simulink model "testBCIRobot"  (Simulink 10.0)
settings: Solver=FixedStepDiscrete  StartTime=0.0  StopTime=inf  FixedStep=0.002  MaxStep=0.02  RelTol=1e-3  AbsTol=1e-6
settings Model: Creator=fwornle  LastModifiedBy=bhisma  ExtModeTrigDuration=5000
settings ConfigSet: Description=rtmc9s12target_R2009b
settings SolverCC: AutoScaleAbsTol=off
settings DataIOCC: SignalLoggingSaveFormat=ModelDataLogs  SaveOutput=off  SaveTime=off  SignalLoggingName=sigsOut
settings OptimizationCC: BlockReduction=off  BooleanDataType=off  ExpressionDepthLimit=2147483647  InitFltsAndDblsToZero=on  LifeSpan=1  EfficientTunableParamExpr=on
settings DebuggingCC: SaveWithParameterizedLinksMsg=none  SignalResolutionControl=TryResolveAllWithWarning  MultiTaskDSMMsg=warning  MultiTaskCondExecSysMsg=none  FcnCallInpInsideContextMsg=warning  StateNameClashWarn=warning
settings HardwareCC: ProdBitPerInt=16  ProdBitPerPointer=16  ProdBitPerSizeT=16  ProdBitPerPtrDiffT=16  ProdEndianess=BigEndian  ProdWordSize=16  ProdHWDeviceType=Motorola HC12
settings SFSimCC: MATLABDynamicMemAlloc=off
settings RTWCC: SystemTargetFile=mc9s12.tlc  GenerateMakefile=off  TemplateMakefile=mc9s12.tmf
settings CodeAppCC: IgnoreCustomStorageClasses=off  CustomSymbolStrType=$N$R$M  InternalIdentifier=Classic
settings STFCustomTargetCC: TargetFcnLib=ansi_tfl_tmw.mat  ModelReferenceCompliant=off  IncludeMdlTerminateFcn=off  ERTCustomFileBanners=on  SupportNonInlinedSFcns=off  RemoveResetFunc=on  MATLABClassNameForMDSCustomization=Simulink.SoftwareTarget.ERTCustomization  CPPClassGenCompliant=on  SystemTargetFile=mc9s12.tlc
settings ERTTargetCC: TargetFcnLib=ansi_tfl_tmw.mat  MultiwordLength=2048  ModelReferenceCompliant=off  ParMdlRefBuildCompliant=off  CompOptLevelCompliant=off  ConcurrentExecutionCompliant=off  IncludeMdlTerminateFcn=off  CombineOutputUpdateFcns=off  SupportContinuousTime=on  ModelStepFunctionPrototypeControlCompliant=off  GRTInterface=on  UseToolchainInfoCompliant=off  ExtModeMexFile=ext_serial_mc9s12_comm  ExtModeMexArgs=1,2,115200  ERTCustomFileTemplate=mc9s12_file_process.tlc  ConvertIfToSwitch=off  SuppressUnreachableDefaultCases=off
settings CustomProperty: DataType=RTWOptions_EnumType_C__Users_fw__SVN_rtmc9s12-target_trunk_rtmc9s12_CW_R2009b_bin_mc9s12_1mc9s12_TargetBoard  Value=MiniDragonPlus-RevE
settings EnumStrPairs: String=Dragon12
settings ConfigComp: CovExternalEMLEnable=off

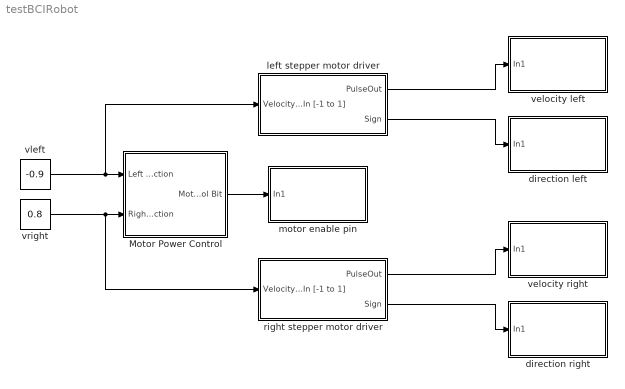
== system testBCIRobot ==
  Motor Power Control : Subsystem
  direction left : Subsystem  Tag=mcTarget_digOut  mask{port=Port A, pin=5, sampletime=0.002, Von=0.5, Voff=0.5}
      mask prompts: port "Port (see hardware manuals for valid options)"; pin "Pin (see hardware manuals for valid options)"; sampletime "Sample time"; Von "On-threshold (Von)"; Voff "Off-threshold (Voff)"
      mask init:
      | [portstr, pinstr, pins] = mbc_digitaloutput(port, pin, sampletime, Von, Voff);
      mask Help: web('digOut_sfcn_9S12.html');
      mask TypeOptions port: Port A | Port B | Port H | Port J | Port M | Port P | Port S | Port T
      mask Display: fprintf('%s\nPins: %s', portstr, pinstr)
  direction right : Subsystem  Tag=mcTarget_digOut  mask{port=Port A, pin=7, sampletime=0.002, Von=0.5, Voff=0.5}
      mask prompts: port "Port (see hardware manuals for valid options)"; pin "Pin (see hardware manuals for valid options)"; sampletime "Sample time"; Von "On-threshold (Von)"; Voff "Off-threshold (Voff)"
      mask init:
      | [portstr, pinstr, pins] = mbc_digitaloutput(port, pin, sampletime, Von, Voff);
      mask Help: web('digOut_sfcn_9S12.html');
      mask TypeOptions port: Port A | Port B | Port H | Port J | Port M | Port P | Port S | Port T
      mask Display: fprintf('%s\nPins: %s', portstr, pinstr)
  left stepper motor driver : Subsystem  mask{Nmax=200, Ninc=20, Ts=2e-3}
      mask prompts: Nmax "Maximum number of pulses per second (Nmax)"; Ninc "Number of increments (Ninc = 1 ... Nmax)"; Ts "Sample time"
      mask help: The block sample time (seconds) is used to clock the digital motor driver algorithm. Smaller values lead to slower pulse sequences.
      mask init:
      | Nmax = floor(abs(Nmax));
      | Ninc = max(1, floor(abs(Ninc)));
      | if (Ninc > Nmax)
      | 	error(['Stepper motor driver: Invalid number of increments (Ninc = ' num2str(Ninc) '; value must be smaller or equal to Nmax = ' num2str(Nmax) ')'])
      | end
      | 
      | % work out pulse length
      | Tpulse_ = 1/Nmax/2;
      | %disp(['Pulse length: ' num2str(1000*Tpulse_) ' ms.'])
      | 
      | % ensure that sample time is fixed multiple of 'Ts'
      | Tpulse = ceil(Tpulse_/Ts)*Ts;
      | if (Tpulse > Tpulse_)
      | 	disp('Decreasing maximum number of pulses per second to ensure that the pulse duration is an integer multiple of ''Ts''')
      | 	
      | 	% adjust Nmax
      | 	Nmax = floor(1/Tpulse/2);
      | 	disp(['New Nmax: ' num2str(Nmax) ' pulses per second.'])
      | end
      | 	
      | % work out quantization interval
      | dQ = floor(Nmax/Ninc);
  motor enable pin : Subsystem  Tag=mcTarget_digOut  mask{port=Port T, pin=7, sampletime=0.002, Von=0.5, Voff=0.5}
      mask prompts: port "Port (see hardware manuals for valid options)"; pin "Pin (see hardware manuals for valid options)"; sampletime "Sample time"; Von "On-threshold (Von)"; Voff "Off-threshold (Voff)"
      mask init:
      | [portstr, pinstr, pins] = mbc_digitaloutput(port, pin, sampletime, Von, Voff);
      mask Help: web('digOut_sfcn_9S12.html');
      mask TypeOptions port: Port A | Port B | Port H | Port J | Port M | Port P | Port S | Port T
      mask Display: fprintf('%s\nPins: %s', portstr, pinstr)
  right stepper motor driver : Subsystem  mask{Nmax=200, Ninc=20, Ts=2e-3}
      mask prompts: Nmax "Maximum number of pulses per second (Nmax)"; Ninc "Number of increments (Ninc = 1 ... Nmax)"; Ts "Sample time"
      mask help: The block sample time (seconds) is used to clock the digital motor driver algorithm. Smaller values lead to slower pulse sequences.
      mask init: same as testBCIRobot/left stepper motor driver
  velocity left : Subsystem  Tag=mcTarget_digOut  mask{port=Port A, pin=4, sampletime=0.002, Von=0.5, Voff=0.5}
      mask prompts: port "Port (see hardware manuals for valid options)"; pin "Pin (see hardware manuals for valid options)"; sampletime "Sample time"; Von "On-threshold (Von)"; Voff "Off-threshold (Voff)"
      mask init:
      | [portstr, pinstr, pins] = mbc_digitaloutput(port, pin, sampletime, Von, Voff);
      mask Help: web('digOut_sfcn_9S12.html');
      mask TypeOptions port: Port A | Port B | Port H | Port J | Port M | Port P | Port S | Port T
      mask Display: fprintf('%s\nPins: %s', portstr, pinstr)
  velocity right : Subsystem  Tag=mcTarget_digOut  mask{port=Port A, pin=6, sampletime=0.002, Von=0.5, Voff=0.5}
      mask prompts: port "Port (see hardware manuals for valid options)"; pin "Pin (see hardware manuals for valid options)"; sampletime "Sample time"; Von "On-threshold (Von)"; Voff "Off-threshold (Voff)"
      mask init:
      | [portstr, pinstr, pins] = mbc_digitaloutput(port, pin, sampletime, Von, Voff);
      mask Help: web('digOut_sfcn_9S12.html');
      mask TypeOptions port: Port A | Port B | Port H | Port J | Port M | Port P | Port S | Port T
      mask Display: fprintf('%s\nPins: %s', portstr, pinstr)
  vleft : Constant  Value=-0.9
  vright : Constant  Value=0.8
  wires:
  left stepper motor driver/1(PulseOut) -> velocity left/1(In1)
  left stepper motor driver/2(Sign) -> direction left/1(In1)
  right stepper motor driver/1(PulseOut) -> velocity right/1(In1)
  right stepper motor driver/2(Sign) -> direction right/1(In1)
  Motor Power Control/1(Motor Control Bit) -> motor enable pin/1(In1)
  vleft/1 -> Motor Power Control/1(Left Motor Instruction), left stepper motor driver/1(VelocityIn [-1 to 1])
  vright/1 -> Motor Power Control/2(Right Motor  Instruction), right stepper motor driver/1(VelocityIn [-1 to 1])

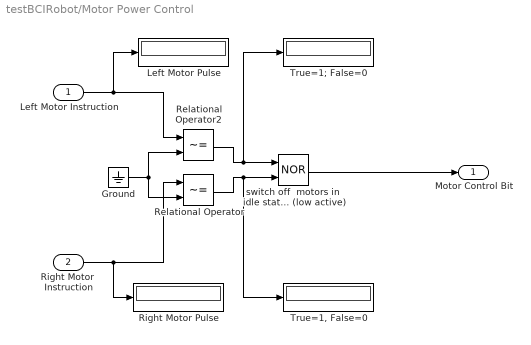
== system testBCIRobot/Motor Power Control ==
  Left Motor Instruction : Inport
  Right Motor  Instruction : Inport  Port=2
  Ground : Ground
  Left Motor Pulse : Display
  Relational Operator : RelationalOperator  Operator=~=  RndMeth=Nearest
  Relational Operator2 : RelationalOperator  Operator=~=  RndMeth=Nearest
  Right Motor Pulse : Display
  "True=1, False=0" : Display
  True=1; False=0 : Display
  switch off  motors in  idle state (low active) : Logic  Operator=NOR  AllPortsSameDT=off
  Motor Control Bit : Outport
  wires:
  Right Motor  Instruction/1 -> Relational Operator/1, Right Motor Pulse/1
  Left Motor Instruction/1 -> Relational Operator2/1, Left Motor Pulse/1
  Ground/1 -> Relational Operator2/2, Relational Operator/2
  Relational Operator2/1 -> switch off  motors in  idle state (low active)/1, True=1; False=0/1
  Relational Operator/1 -> switch off  motors in  idle state (low active)/2, "True=1, False=0"/1
  switch off  motors in  idle state (low active)/1 -> Motor Control Bit/1

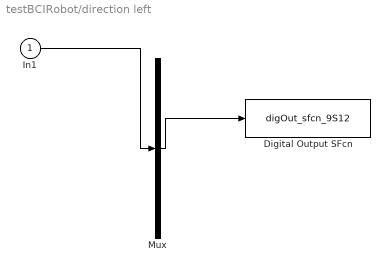
== system testBCIRobot/direction left ==
  In1 : Inport
  Digital Output SFcn : S-Function  Tag=mcTarget_digOut  FunctionName=digOut_sfcn_9S12  Parameters=sampletime, port, pins, Von, Voff  SFunctionDeploymentMode=off  EnableBusSupport=off
  Mux : Mux  Inputs=1
  wires:
  In1/1 -> Mux/1
  Mux/1 -> Digital Output SFcn/1

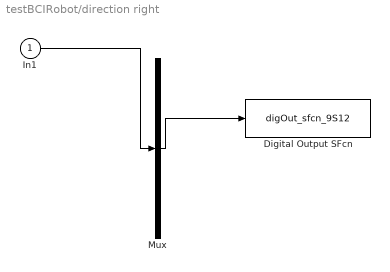
== system testBCIRobot/direction right ==
  In1 : Inport
  Digital Output SFcn : S-Function  Tag=mcTarget_digOut  FunctionName=digOut_sfcn_9S12  Parameters=sampletime, port, pins, Von, Voff  SFunctionDeploymentMode=off  EnableBusSupport=off
  Mux : Mux  Inputs=1
  wires:
  In1/1 -> Mux/1
  Mux/1 -> Digital Output SFcn/1

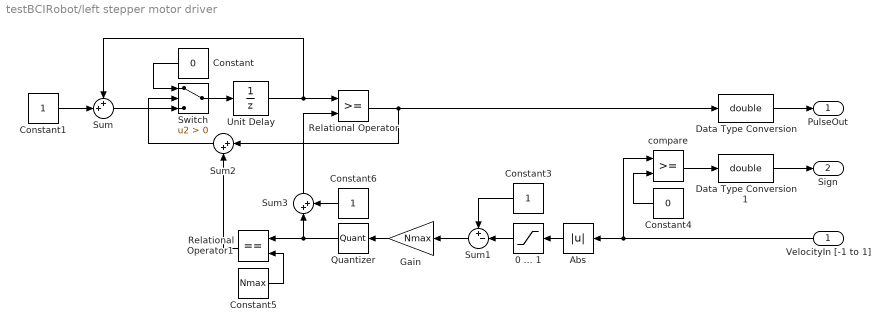
== system testBCIRobot/left stepper motor driver ==
  VelocityIn [-1 to 1] : Inport
  0 ... 1 : Saturate  UpperLimit=1  LowerLimit=0
  Abs : Abs
  Constant : Constant  Value=0
  Constant1 : Constant
  Constant3 : Constant
  Constant4 : Constant  Value=0
  Constant5 : Constant  Value=Nmax
  Constant6 : Constant
  Data Type Conversion : DataTypeConversion  OutDataTypeStr=double  SaturateOnIntegerOverflow=on  RndMeth=Zero
  Data Type Conversion1 : DataTypeConversion  OutDataTypeStr=double  SaturateOnIntegerOverflow=on  RndMeth=Zero
  Gain : Gain  Gain=Nmax  SaturateOnIntegerOverflow=on  OutDataTypeStr=Inherit: Same as input  ParamDataTypeStr=Inherit: Same as input
  Quantizer : Quantizer  QuantizationInterval=dQ
  Relational Operator : RelationalOperator  OutDataTypeStr=uint(8)  RndMeth=Nearest
  Relational Operator1 : RelationalOperator  Operator===  OutDataTypeStr=uint(8)  RndMeth=Nearest
  Sum : Sum  Inputs=++|
  Sum1 : Sum  Inputs=+-|
  Sum2 : Sum  Inputs=|++
  Sum3 : Sum  Inputs=|++
  Switch : Switch  Criteria=u2 > Threshold
  Unit Delay : UnitDelay  SampleTime=Tpulse
  compare : RelationalOperator  OutDataTypeStr=uint(8)  RndMeth=Nearest
  PulseOut : Outport
  Sign : Outport  Port=2
  wires:
  Constant1/1 -> Sum/2
  Sum3/1 -> Relational Operator/2
  Constant6/1 -> Sum3/2
  Relational Operator1/1 -> Sum2/2
  Sum2/1 -> Switch/2
  Constant5/1 -> Relational Operator1/2
  0 ... 1/1 -> Sum1/2
  Sum1/1 -> Gain/1
  Abs/1 -> 0 ... 1/1
  Constant3/1 -> Sum1/1
  VelocityIn [-1 to 1]/1 -> compare/1, Abs/1
  Gain/1 -> Quantizer/1
  Quantizer/1 -> Sum3/1, Relational Operator1/1
  Constant4/1 -> compare/2
  compare/1 -> Data Type Conversion1/1
  Constant/1 -> Switch/1
  Sum/1 -> Switch/3
  Relational Operator/1 -> Sum2/1, Data Type Conversion/1
  Unit Delay/1 -> Sum/1, Relational Operator/1
  Switch/1 -> Unit Delay/1
  Data Type Conversion/1 -> PulseOut/1
  Data Type Conversion1/1 -> Sign/1

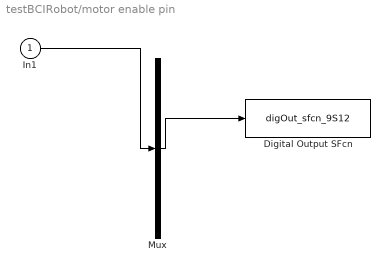
== system testBCIRobot/motor enable pin ==
  In1 : Inport
  Digital Output SFcn : S-Function  Tag=mcTarget_digOut  FunctionName=digOut_sfcn_9S12  Parameters=sampletime, port, pins, Von, Voff  SFunctionDeploymentMode=off  EnableBusSupport=off
  Mux : Mux  Inputs=1
  wires:
  In1/1 -> Mux/1
  Mux/1 -> Digital Output SFcn/1

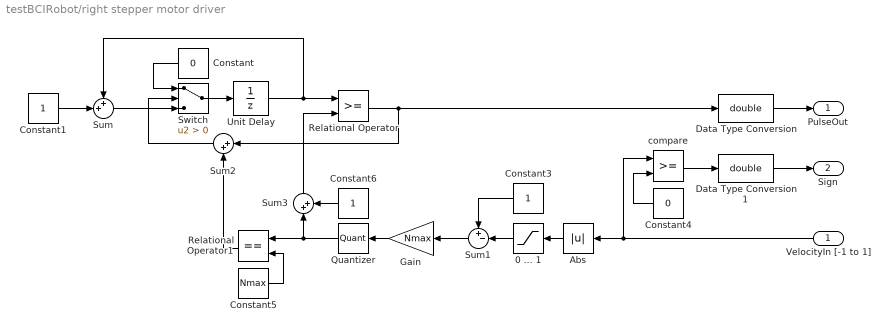
== system testBCIRobot/right stepper motor driver ==
  VelocityIn [-1 to 1] : Inport
  0 ... 1 : Saturate  UpperLimit=1  LowerLimit=0
  Abs : Abs
  Constant : Constant  Value=0
  Constant1 : Constant
  Constant3 : Constant
  Constant4 : Constant  Value=0
  Constant5 : Constant  Value=Nmax
  Constant6 : Constant
  Data Type Conversion : DataTypeConversion  OutDataTypeStr=double  SaturateOnIntegerOverflow=on  RndMeth=Zero
  Data Type Conversion1 : DataTypeConversion  OutDataTypeStr=double  SaturateOnIntegerOverflow=on  RndMeth=Zero
  Gain : Gain  Gain=Nmax  SaturateOnIntegerOverflow=on  OutDataTypeStr=Inherit: Same as input  ParamDataTypeStr=Inherit: Same as input
  Quantizer : Quantizer  QuantizationInterval=dQ
  Relational Operator : RelationalOperator  OutDataTypeStr=uint(8)  RndMeth=Nearest
  Relational Operator1 : RelationalOperator  Operator===  OutDataTypeStr=uint(8)  RndMeth=Nearest
  Sum : Sum  Inputs=++|
  Sum1 : Sum  Inputs=+-|
  Sum2 : Sum  Inputs=|++
  Sum3 : Sum  Inputs=|++
  Switch : Switch  Criteria=u2 > Threshold
  Unit Delay : UnitDelay  SampleTime=Tpulse
  compare : RelationalOperator  OutDataTypeStr=uint(8)  RndMeth=Nearest
  PulseOut : Outport
  Sign : Outport  Port=2
  wires:
  Data Type Conversion1/1 -> Sign/1
  Data Type Conversion/1 -> PulseOut/1
  Switch/1 -> Unit Delay/1
  Unit Delay/1 -> Relational Operator/1, Sum/1
  Relational Operator/1 -> Data Type Conversion/1, Sum2/1
  Sum/1 -> Switch/3
  Constant/1 -> Switch/1
  compare/1 -> Data Type Conversion1/1
  Constant4/1 -> compare/2
  Quantizer/1 -> Relational Operator1/1, Sum3/1
  Gain/1 -> Quantizer/1
  VelocityIn [-1 to 1]/1 -> Abs/1, compare/1
  Constant3/1 -> Sum1/1
  Abs/1 -> 0 ... 1/1
  Sum1/1 -> Gain/1
  0 ... 1/1 -> Sum1/2
  Constant5/1 -> Relational Operator1/2
  Sum2/1 -> Switch/2
  Relational Operator1/1 -> Sum2/2
  Constant6/1 -> Sum3/2
  Sum3/1 -> Relational Operator/2
  Constant1/1 -> Sum/2

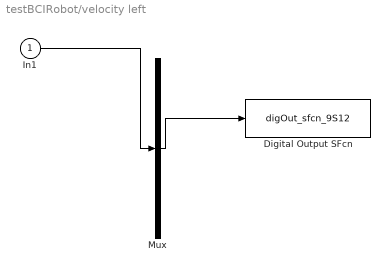
== system testBCIRobot/velocity left ==
  In1 : Inport
  Digital Output SFcn : S-Function  Tag=mcTarget_digOut  FunctionName=digOut_sfcn_9S12  Parameters=sampletime, port, pins, Von, Voff  SFunctionDeploymentMode=off  EnableBusSupport=off
  Mux : Mux  Inputs=1
  wires:
  Mux/1 -> Digital Output SFcn/1
  In1/1 -> Mux/1

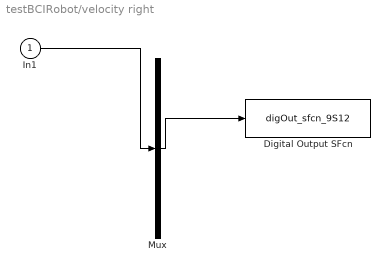
== system testBCIRobot/velocity right ==
  In1 : Inport
  Digital Output SFcn : S-Function  Tag=mcTarget_digOut  FunctionName=digOut_sfcn_9S12  Parameters=sampletime, port, pins, Von, Voff  SFunctionDeploymentMode=off  EnableBusSupport=off
  Mux : Mux  Inputs=1
  wires:
  Mux/1 -> Digital Output SFcn/1
  In1/1 -> Mux/1
